simulink model "sliding_car"  (R2017a)
settings: Solver=VariableStepAuto  StartTime=0.0  StopTime=tf  RelTol=1e-3
values from neighbouring files (symbols this model uses):
  a = double(perc*D)    [init_vars.m]
  Cp_1 = 0    [init_vars.m]
  Cp_2 = 0    [init_vars.m]
  Fz_1 = g*(mc/4 + mi)    [init_vars.m]
  Fz_2 = g*(mc/4 + mi)    [init_vars.m]
  mu_1 = 1e-3    (= 0.001)    [init_vars.m]
  mu_2 = 1e-3    (= 0.001)    [init_vars.m]
  x0 = double(subs([qs; ps], [sys.descrip.syms.'; delta_i],                   [sys.descrip.model_params.'; delta_i_num]))    [init_vars.m]    (also in sim_blockdiagram.m)
undefined symbols (not defined in the file or in its folder): g, Ic_33, Ii_11, Ii_21, Ii_22, Ii_31, Ii_32, Ii_33, Il_11, Il_21, Il_22, Il_31, Il_32, Il_33, Io_11, Io_21, Io_22, Io_31, Io_32, Io_33, Ir_11, Ir_21, Ir_22, Ir_31, Ir_32, Ir_33, L, Lc, mc, mi, ml, mo, mr, R, sys, w
(part 1 of 5)
settings Model: SimulationMode=rapid-accelerator  Creator=brunolnetto  LastModifiedBy=brunolnetto

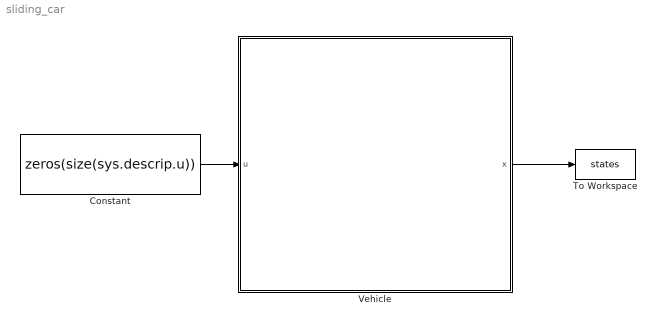
== system sliding_car ==
  Constant : Constant  Value=zeros(size(sys.descrip.u))
  To Workspace : ToWorkspace  VariableName=states  SaveFormat=Structure With Time  SampleTime=-1
  Vehicle : Subsystem
      mask Display: image('/home/brunolnetto/Pictures/auto_model.png');
  wires:
  Constant/1 -> Vehicle/1(u)
  Vehicle/1(x) -> To Workspace/1

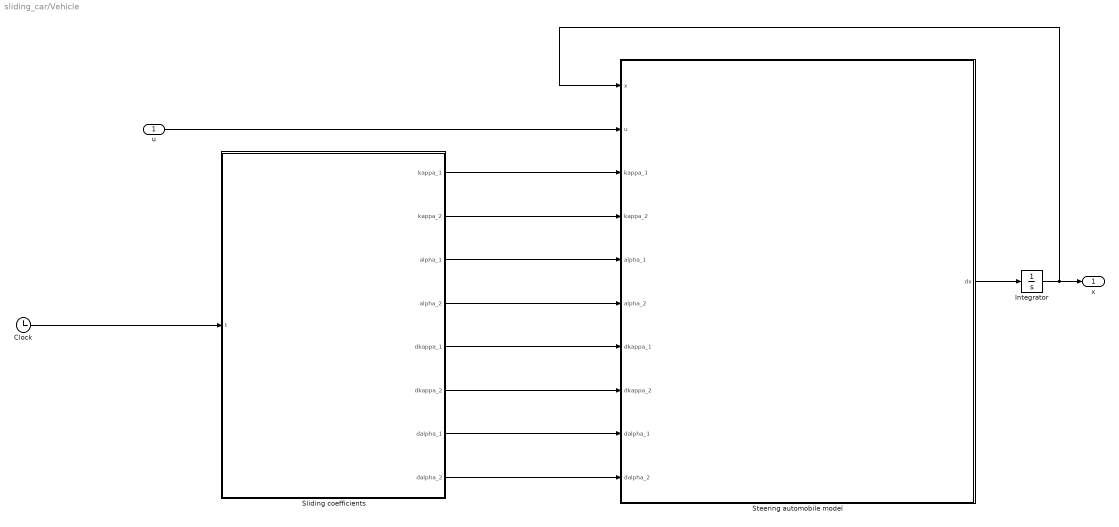
== system sliding_car/Vehicle ==
  u : Inport
  Clock : Clock
  Integrator : Integrator  InitialCondition=x0
  Sliding coefficients : MATLAB Function  TreatAsAtomicUnit=on
  Steering automobile model : Subsystem
      mask Display: image('/home/brunolnetto/Pictures/steer_schema.png');
  x : Outport
  wires:
  Steering automobile model/1(dx) -> Integrator/1
  Sliding coefficients/4(alpha_2) -> Steering automobile model/6(alpha_2)
  Sliding coefficients/3(alpha_1) -> Steering automobile model/5(alpha_1)
  Sliding coefficients/2(kappa_2) -> Steering automobile model/4(kappa_2)
  Sliding coefficients/1(kappa_1) -> Steering automobile model/3(kappa_1)
  u/1 -> Steering automobile model/2(u)
  Clock/1 -> Sliding coefficients/1(t)
  Sliding coefficients/8(dalpha_2) -> Steering automobile model/10(dalpha_2)
  Sliding coefficients/7(dalpha_1) -> Steering automobile model/9(dalpha_1)
  Sliding coefficients/6(dkappa_2) -> Steering automobile model/8(dkappa_2)
  Sliding coefficients/5(dkappa_1) -> Steering automobile model/7(dkappa_1)
  Integrator/1 -> Steering automobile model/1(x), x/1

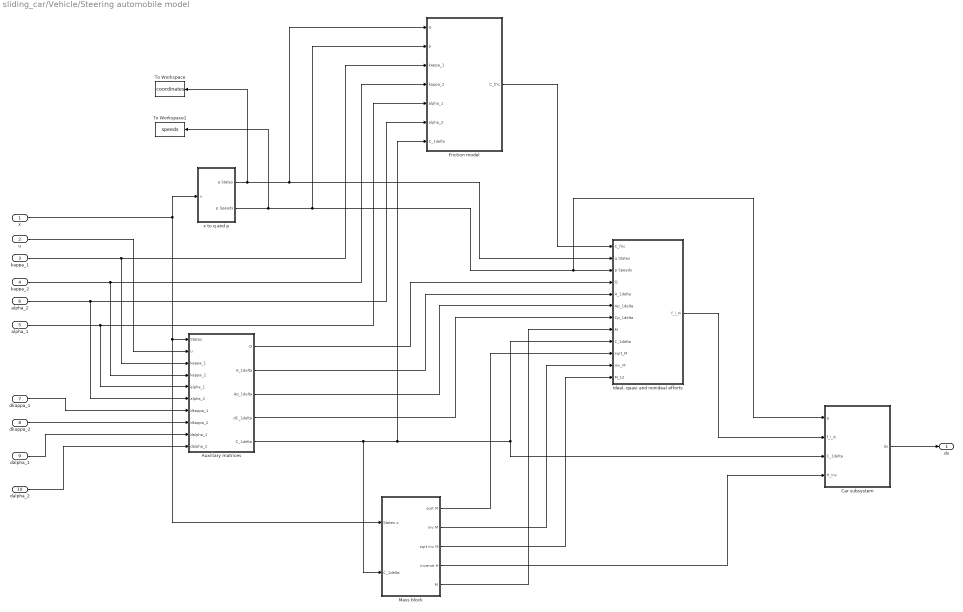
== system sliding_car/Vehicle/Steering automobile model ==
  x : Inport
  u : Inport  Port=2
  kappa_1 : Inport  Port=3
  kappa_2 : Inport  Port=4
  alpha_1 : Inport  Port=5
  alpha_2 : Inport  Port=6
  dkappa_1 : Inport  Port=7
  dkappa_2 : Inport  Port=8
  dalpha_1 : Inport  Port=9
  dalpha_2 : Inport  Port=10
  Auxiliary matrices : Subsystem
  Car subsystem : Subsystem
  Friction model : MATLAB Function  TreatAsAtomicUnit=on
  "Ideal, quasi and nonideal efforts" : Subsystem
  Mass block : Subsystem
  To Workspace : ToWorkspace  VariableName=coordinates  SaveFormat=Structure With Time  SampleTime=-1
  To Workspace1 : ToWorkspace  VariableName=speeds  SaveFormat=Structure With Time  SampleTime=-1
  x to q and p : Subsystem
  dx : Outport
  wires:
  kappa_1/1 -> Auxiliary matrices/3(kappa_1), Friction model/3(kappa_1)
  alpha_2/1 -> Auxiliary matrices/6(alpha_2), Friction model/6(alpha_2)
  alpha_1/1 -> Friction model/5(alpha_1), Auxiliary matrices/5(alpha_1)
  x/1 -> x to q and p/1(x), Mass block/1(States x), Auxiliary matrices/1(States)
  Auxiliary matrices/5("C_1delta ") -> Friction model/7(C_1delta), "Ideal, quasi and nonideal efforts"/9(C_1delta), Car subsystem/3(C_1delta), Mass block/2("C_1delta  ")
  u/1 -> Auxiliary matrices/2(u)
  Auxiliary matrices/1("Q ") -> "Ideal, quasi and nonideal efforts"/4(Q)
  Auxiliary matrices/2("A_1delta ") -> "Ideal, quasi and nonideal efforts"/5(A_1delta)
  Auxiliary matrices/3("Ap_1delta ") -> "Ideal, quasi and nonideal efforts"/6(Ap_1delta)
  Auxiliary matrices/4("dC_1delta ") -> "Ideal, quasi and nonideal efforts"/7(Cp_1delta)
  Mass block/1(sqrt M) -> "Ideal, quasi and nonideal efforts"/10(sqrt_M)
  Mass block/2(inv M) -> "Ideal, quasi and nonideal efforts"/11(inv_M)
  Mass block/3(sqrt inv M) -> "Ideal, quasi and nonideal efforts"/12(M_12)
  dalpha_1/1 -> Auxiliary matrices/9(dalpha_1)
  dkappa_2/1 -> Auxiliary matrices/8(dkappa_2)
  dalpha_2/1 -> Auxiliary matrices/10(dalpha_2)
  dkappa_1/1 -> Auxiliary matrices/7(dkappa_1)
  Mass block/5(M) -> "Ideal, quasi and nonideal efforts"/8(M)
  kappa_2/1 -> Auxiliary matrices/4(kappa_2), Friction model/4(kappa_2)
  Friction model/1(C_fric) -> "Ideal, quasi and nonideal efforts"/1(C_fric)
  Mass block/4(inverse H) -> Car subsystem/4(H_inv)
  Car subsystem/1(dx) -> dx/1
  "Ideal, quasi and nonideal efforts"/1(f_i_ni) -> Car subsystem/2(f_i_ni)
  x to q and p/1(q States) -> Friction model/1(q), "Ideal, quasi and nonideal efforts"/2(q States), To Workspace/1
  x to q and p/2(p Speeds) -> To Workspace1/1, Friction model/2(p), Car subsystem/1(p), "Ideal, quasi and nonideal efforts"/3(p Speeds)

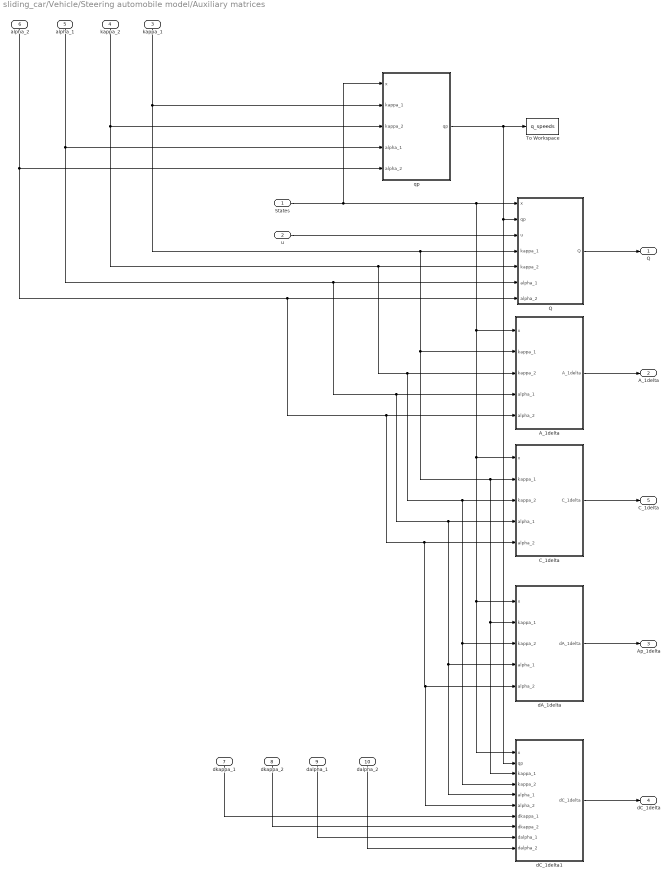
== system sliding_car/Vehicle/Steering automobile model/Auxiliary matrices ==
  States : Inport
  u : Inport  Port=2
  kappa_1 : Inport  Port=3
  kappa_2 : Inport  Port=4
  alpha_1 : Inport  Port=5
  alpha_2 : Inport  Port=6
  dkappa_1 : Inport  Port=7
  dkappa_2 : Inport  Port=8
  dalpha_1 : Inport  Port=9
  dalpha_2 : Inport  Port=10
  A_1delta : MATLAB Function  TreatAsAtomicUnit=on
  C_1delta : MATLAB Function  TreatAsAtomicUnit=on
  Q : MATLAB Function  TreatAsAtomicUnit=on
  To Workspace : ToWorkspace  VariableName=q_speeds  SaveFormat=Structure With Time  SampleTime=-1
  dA_1delta : MATLAB Function  TreatAsAtomicUnit=on
  dC_1delta1 : MATLAB Function  TreatAsAtomicUnit=on
  qp : MATLAB Function  TreatAsAtomicUnit=on
  "Q " : Outport
  "A_1delta " : Outport  Port=2
  "Ap_1delta " : Outport  Port=3
  "dC_1delta " : Outport  Port=4
  "C_1delta " : Outport  Port=5
  wires:
  alpha_2/1 -> Q/7(alpha_2), A_1delta/5(alpha_2), dC_1delta1/6(alpha_2), dA_1delta/5(alpha_2), C_1delta/5(alpha_2), qp/5(alpha_2)
  kappa_2/1 -> Q/5(kappa_2), A_1delta/3(kappa_2), dC_1delta1/4(kappa_2), dA_1delta/3(kappa_2), C_1delta/3(kappa_2), qp/3(kappa_2)
  kappa_1/1 -> A_1delta/2(kappa_1), dC_1delta1/3(kappa_1), dA_1delta/2(kappa_1), C_1delta/2(kappa_1), Q/4(kappa_1), qp/2(kappa_1)
  C_1delta/1(C_1delta) -> "C_1delta "/1
  Q/1(Q) -> "Q "/1
  A_1delta/1(A_1delta) -> "A_1delta "/1
  dC_1delta1/1(dC_1delta) -> "dC_1delta "/1
  dA_1delta/1(dA_1delta) -> "Ap_1delta "/1
  u/1 -> Q/3(u)
  alpha_1/1 -> Q/6(alpha_1), dC_1delta1/5(alpha_1), dA_1delta/4(alpha_1), C_1delta/4(alpha_1), A_1delta/4(alpha_1), qp/4(alpha_1)
  States/1 -> qp/1(x), A_1delta/1(x), dC_1delta1/1(x), dA_1delta/1(x), C_1delta/1(x), Q/1(x)
  qp/1(qp) -> To Workspace/1, dC_1delta1/2(qp), Q/2(qp)
  dalpha_2/1 -> dC_1delta1/10(dalpha_2)
  dalpha_1/1 -> dC_1delta1/9(dalpha_1)
  dkappa_2/1 -> dC_1delta1/8(dkappa_2)
  dkappa_1/1 -> dC_1delta1/7(dkappa_1)

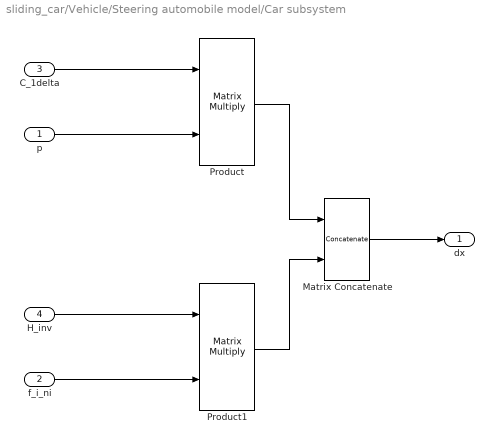
== system sliding_car/Vehicle/Steering automobile model/Car subsystem ==
  p : Inport
  f_i_ni : Inport  Port=2
  C_1delta : Inport  Port=3
  H_inv : Inport  Port=4
  Matrix Concatenate : Concatenate  ConcatenateDimension=2
  Product : Product  Multiplication=Matrix(*)
  Product1 : Product  Multiplication=Matrix(*)
  dx : Outport
  wires:
  Product/1 -> Matrix Concatenate/1
  p/1 -> Product/2
  C_1delta/1 -> Product/1
  Product1/1 -> Matrix Concatenate/2
  H_inv/1 -> Product1/1
  f_i_ni/1 -> Product1/2
  Matrix Concatenate/1 -> dx/1

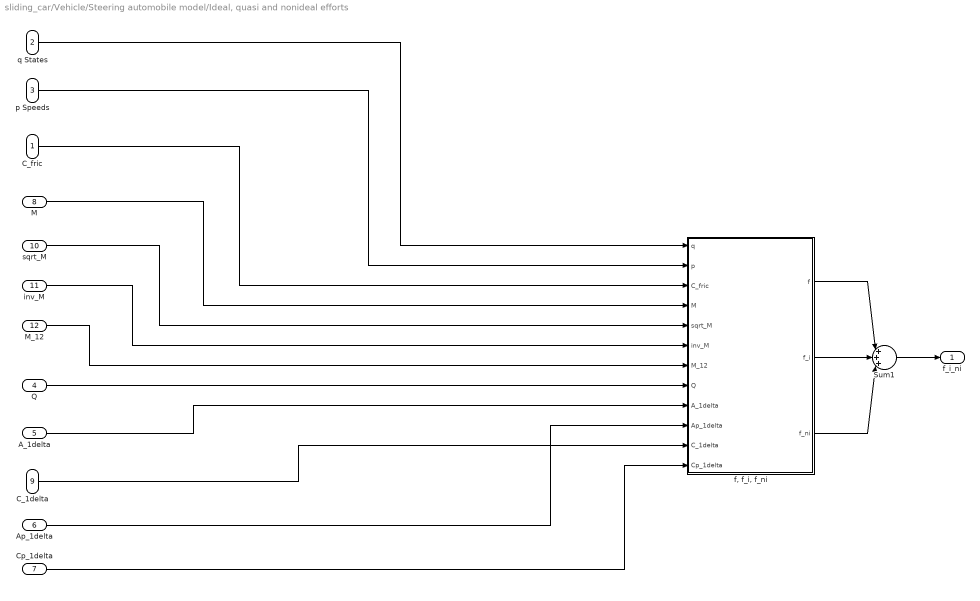
== system sliding_car/Vehicle/Steering automobile model/Ideal, quasi and nonideal efforts ==
  C_fric : Inport
  q States : Inport  Port=2
  p Speeds : Inport  Port=3
  Q : Inport  Port=4
  A_1delta : Inport  Port=5
  Ap_1delta : Inport  Port=6
  Cp_1delta : Inport  Port=7
  M : Inport  Port=8
  C_1delta : Inport  Port=9
  sqrt_M : Inport  Port=10
  inv_M : Inport  Port=11
  M_12 : Inport  Port=12
  Sum1 : Sum  Inputs=|+++|
  "f, f_i, f_ni" : MATLAB Function  TreatAsAtomicUnit=on
  f_i_ni : Outport
  wires:
  inv_M/1 -> "f, f_i, f_ni"/6(inv_M)
  sqrt_M/1 -> "f, f_i, f_ni"/5(sqrt_M)
  M_12/1 -> "f, f_i, f_ni"/7(M_12)
  C_1delta/1 -> "f, f_i, f_ni"/11(C_1delta)
  Q/1 -> "f, f_i, f_ni"/8(Q)
  A_1delta/1 -> "f, f_i, f_ni"/9(A_1delta)
  Cp_1delta/1 -> "f, f_i, f_ni"/12(Cp_1delta)
  Ap_1delta/1 -> "f, f_i, f_ni"/10(Ap_1delta)
  C_fric/1 -> "f, f_i, f_ni"/3(C_fric)
  M/1 -> "f, f_i, f_ni"/4(M)
  q States/1 -> "f, f_i, f_ni"/1(q)
  p Speeds/1 -> "f, f_i, f_ni"/2(p)
  "f, f_i, f_ni"/1(f) -> Sum1/1
  Sum1/1 -> f_i_ni/1
  "f, f_i, f_ni"/2(f_i) -> Sum1/2
  "f, f_i, f_ni"/3(f_ni) -> Sum1/3

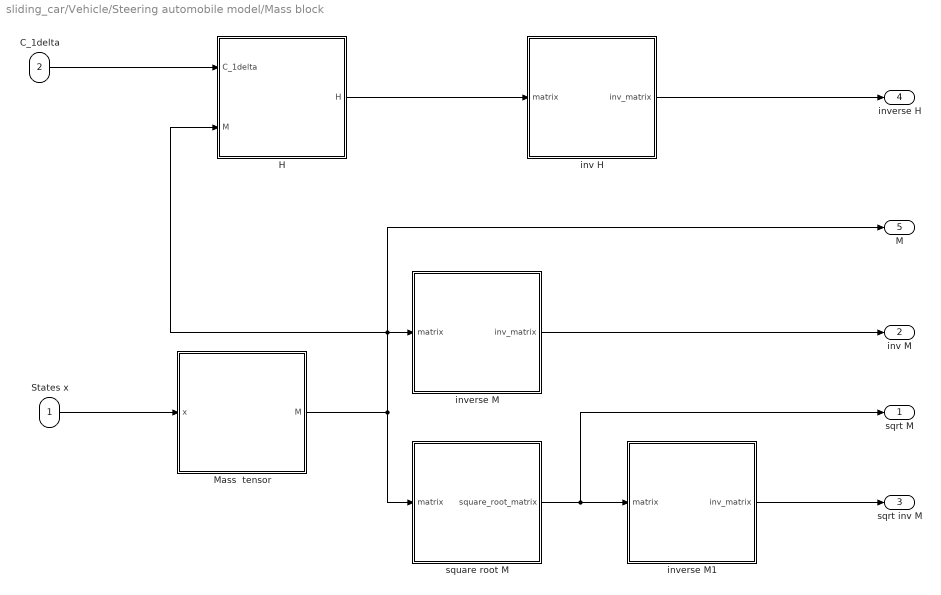
== system sliding_car/Vehicle/Steering automobile model/Mass block ==
  States x : Inport
  "C_1delta  " : Inport  Port=2
  H : MATLAB Function  TreatAsAtomicUnit=on
  Mass  tensor : MATLAB Function  TreatAsAtomicUnit=on
  inv H : MATLAB Function  TreatAsAtomicUnit=on
  inverse M : MATLAB Function  TreatAsAtomicUnit=on
  inverse M1 : MATLAB Function  TreatAsAtomicUnit=on
  square root M : MATLAB Function  TreatAsAtomicUnit=on
  sqrt M : Outport
  inv M : Outport  Port=2
  sqrt inv M : Outport  Port=3
  inverse H : Outport  Port=4
  M : Outport  Port=5
  wires:
  States x/1 -> Mass  tensor/1(x)
  "C_1delta  "/1 -> H/1(C_1delta)
  inverse M/1(inv_matrix) -> inv M/1
  H/1(H) -> inv H/1(matrix)
  inv H/1(inv_matrix) -> inverse H/1
  inverse M1/1(inv_matrix) -> sqrt inv M/1
  Mass  tensor/1(M) -> M/1, H/2(M), inverse M/1(matrix), square root M/1(matrix)
  square root M/1(square_root_matrix) -> sqrt M/1, inverse M1/1(matrix)

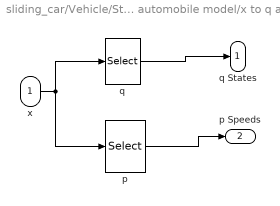
== system sliding_car/Vehicle/Steering automobile model/x to q and p ==
  x : Inport
  p : Selector  InputPortWidth=12  IndexOptions=Index vector (dialog)  Indices=[10 11 12]  OutputSizes=1
  q : Selector  InputPortWidth=12  IndexOptions=Index vector (dialog)  Indices=[1 2 3 4 5 6 7 8 9]  OutputSizes=1
  q States : Outport
  p Speeds : Outport  Port=2
  wires:
  x/1 -> p/1, q/1
  q/1 -> q States/1
  p/1 -> p Speeds/1

== matlab function sliding_car/Vehicle/Steering automobile model/Auxiliary matrices/A_1delta ==
  data: x input; kappa_1 input; kappa_2 input; alpha_1 input; alpha_2 input; w parameter; A_1delta output; L parameter; R parameter
function A_1delta = ConstraintMatrix(x, kappa_1, kappa_2, alpha_1, alpha_2, w, L, R)
%CONSTRAINTMATRIX
%    A_1DELTA = CONSTRAINTMATRIX(L,R,ALPHA_1,ALPHA_2,DELTA_I,DELTA_O,KAPPA_1,KAPPA_2,THETA,W)

%    This function was generated by the Symbolic Math Toolbox version 7.2.
%    16-Oct-2020 13:31:39
    
    x_pos =  x(1);
    y_pos =  x(2);
    theta =  x(3);

    delta_i = x(4);
    delta_o = x(5);

    phi_i = x(6);
    phi_l = x(7);
    phi_o = x(8);
    phi_r = x(9);

    t2 = tan(delta_i);
    t3 = 1.0./L;
    t4 = t2.*w;
    t5 = L+t4;
    t6 = 1.0./t5;
    t7 = t2.*t6;
    t8 = tan(t7);
    t9 = delta_i+theta;
    t10 = cos(t9);
    t11 = sin(t9);
    t12 = tan(alpha_1);
    t13 = cos(delta_i);
    t14 = sin(delta_i);
    t15 = t14.*w.*(1.0./2.0);
    t16 = kappa_1.*t10.*t12;
    t17 = kappa_1.*t11.*t12;
    t18 = kappa_1.*t12.*(t15-L.*t13);
    t19 = L.*t8;
    t20 = atan(t19);
    t21 = t20+theta;
    t22 = delta_o+theta;
    t23 = tan(alpha_2);
    t24 = L.^2;
    t25 = t8.^2;
    t26 = t24.*t25;
    t27 = t26+1.0;
    t28 = 1.0./sqrt(t27);
    t29 = sin(t21);
    t30 = cos(t22);
    t31 = kappa_2.*t23.*t30;
    t32 = cos(t21);
    t33 = sin(t22);
    t34 = kappa_2.*t23.*t33;
    t35 = cos(delta_o);
    t36 = L.*t35;
    t37 = sin(delta_o);
    t38 = t37.*w.*(1.0./2.0);
    t39 = t36+t38;
    A_1delta = reshape([0.0,0.0,t10+t16,-t11+t16,t31+t32,-t29+t31,0.0,0.0, ...
                        t11+t17,t10+t17,t29+t34,t32+t34,0.0,0.0,t15+t18-L.*t13, ...
                        t18+L.*t14+t13.*w.*(1.0./2.0),-L.*t28-kappa_2.*t23.*t39-L.*t8.*t28.*w.*(1.0./2.0), ...
                        t28.*w.*(-1.0./2.0)-kappa_2.*t23.*t39+t8.*t24.*t28,t3.*(t2.^2+1.0).*(L-L.*t8.*w), ...
                        0.0,0.0,0.0,0.0,0.0,-t3.*t5.*t27,0.0,0.0,0.0,0.0,0.0,0.0,0.0,-R,0.0,0.0,0.0, ...
                        0.0,0.0,0.0,0.0,-R,0.0,0.0,-t2.*t3.*w-1.0,0.0,0.0,0.0,0.0,0.0,1.0,0.0,0.0,0.0,0.0],[6,9]);

== matlab function sliding_car/Vehicle/Steering automobile model/Mass block/Mass  tensor ==
  data: x input; M output; Io_32 parameter; Io_33 parameter; Ir_11 parameter; Ir_21 parameter; Ir_22 parameter; Ir_31 parameter; Ir_32 parameter; Ic_33 parameter; Ii_11 parameter; Ii_21 parameter; Ii_22 parameter; Ii_31 parameter; Ii_32 parameter; Ii_33 parameter; Il_11 parameter; Il_21 parameter; Il_22 parameter; Il_31 parameter; Il_32 parameter; Il_33 parameter; Io_11 parameter; Io_21 parameter; Io_22 parameter; Io_31 parameter; Ir_33 parameter; L parameter; Lc parameter; mc parameter; mi parameter; ml parameter; mo parameter; mr parameter; w parameter
function M = MassMatrix(x, ...
                        Io_32, Io_33,...
                        Ir_11, Ir_21, Ir_22, Ir_31, Ir_32, Ic_33, ...
                        Ii_11, Ii_21, Ii_22, Ii_31, Ii_32, Ii_33,...
                        Il_11, Il_21, Il_22, Il_31, Il_32, Il_33,...
                        Io_11, Io_21, Io_22, Io_31, Ir_33,...
                        L, Lc, mc, mi, ml, mo, mr, w)
% MASSMATRIX
%    OUT1 = MASSMATRIX(IC_33,II_11,II_21,II_22,II_31,II_32,II_33,IL_11,IL_21,IL_22,IL_31,IL_32,IL_33,IO_11,IO_21,IO_22,IO_31,IO_32,IO_33,IR_11,IR_21,IR_22,IR_31,IR_32,IR_33,L,LC,DELTA_I,DELTA_O,MC,MI,ML,MO,MR,PHI_I,PHI_L,PHI_O,PHI_R,THETA,W)

%    This function was generated by the Symbolic Math Toolbox version 7.2.
%    16-Oct-2020 11:55:07

x_pos =  x(1);
y_pos =  x(2);
theta =  x(3);

delta_i = x(4);
delta_o = x(5);

phi_i = x(6);
phi_l = x(7);
phi_o = x(8);
phi_r = x(9);

t2 = sin(theta);
t3 = cos(theta);
t4 = mc+mi+ml+mo+mr;
t5 = mo.*t2.*w.*(1.0./2.0);
t6 = mr.*t2.*w.*(1.0./2.0);
t7 = t5+t6-L.*mi.*t3-L.*mo.*t3-Lc.*mc.*t3-mi.*t2.*w.*(1.0./2.0)-ml.*t2.*w.*(1.0./2.0);
t8 = mi.*t3.*w.*(1.0./2.0);
t9 = ml.*t3.*w.*(1.0./2.0);
t10 = t8+t9-L.*mi.*t2-L.*mo.*t2-Lc.*mc.*t2-mo.*t3.*w.*(1.0./2.0)-mr.*t3.*w.*(1.0./2.0);
t11 = cos(phi_i);
t12 = t11.^2;
t13 = cos(phi_l);
t14 = t13.^2;
t15 = cos(phi_o);
t16 = t15.^2;
t17 = cos(phi_r);
t18 = t17.^2;
t19 = sin(phi_l);
t20 = t19.^2;
t21 = t3.^2;
t22 = sin(phi_r);
t23 = t22.^2;
t24 = t2.^2;
t25 = L.^2;
t26 = Lc.^2;
t27 = w.^2;
t28 = t14-1.0;
t29 = t18-1.0;
t30 = cos(delta_i);
t31 = sin(phi_i);
t32 = t31.^2;
t33 = cos(delta_o);
t34 = sin(phi_o);
t35 = t34.^2;
t36 = t30.^2;
t37 = sin(delta_i);
t38 = t33.^2;
t39 = sin(delta_o);
t40 = t37.^2;
t41 = t32.^2;
t42 = t39.^2;
t43 = t35.^2;
t44 = phi_i.*4.0;
t45 = cos(t44);
t46 = t45-1.0;
t47 = t12.^2;
t48 = Ii_33.*t47;
t49 = Ii_33.*t21.*t36.*t41;
t50 = Ii_22.*t24.*t32.*t36;
t51 = Ii_22.*t21.*t32.*t40;
t52 = Ii_33.*t24.*t40.*t41;
t53 = Ii_31.*t11.*t21.*t31.*t32.*t36.*2.0;
t54 = Ii_31.*t11.*t24.*t31.*t32.*t40.*2.0;
t55 = Ii_31.*t3.*t11.*t30.*t31.*t32.*2.0;
t56 = Ii_32.*t2.*t12.*t30.*t31.*2.0;
t57 = Ii_32.*t3.*t12.*t31.*t37.*2.0;
t58 = Ii_11.*t12.*t21.*t32.*t36;
t59 = Ii_31.*t2.*t11.*t12.*t31.*t37.*2.0;
t60 = Ii_11.*t12.*t24.*t32.*t40;
t61 = Ii_11.*t3.*t12.*t30.*t32.*2.0;
t62 = Ii_32.*t24.*t30.*t31.*t32.*t37.*2.0;
t63 = Ii_33.*t2.*t12.*t32.*t37.*2.0;
t64 = Ii_32.*t2.*t3.*t31.*t32.*t40.*2.0;
t65 = Ii_22.*t2.*t3.*t30.*t32.*t37.*2.0;
t66 = Ii_21.*t11.*t24.*t30.*t32.*t37.*2.0;
t67 = Ii_21.*t2.*t3.*t11.*t32.*t40.*2.0;
t68 = phi_o.*4.0;
t69 = cos(t68);
t70 = t69-1.0;
t71 = t16.^2;
t72 = Io_33.*t71;
t73 = Io_33.*t21.*t38.*t43;
t74 = Io_22.*t24.*t35.*t38;
t75 = Io_22.*t21.*t35.*t42;
t76 = Io_33.*t24.*t42.*t43;
t77 = Io_31.*t15.*t21.*t34.*t35.*t38.*2.0;
t78 = Io_31.*t15.*t24.*t34.*t35.*t42.*2.0;
t79 = Io_31.*t3.*t15.*t33.*t34.*t35.*2.0;
t80 = Io_32.*t2.*t16.*t33.*t34.*2.0;
t81 = Io_32.*t3.*t16.*t34.*t39.*2.0;
t82 = Io_11.*t16.*t21.*t35.*t38;
t83 = Io_31.*t2.*t15.*t16.*t34.*t39.*2.0;
t84 = Io_11.*t16.*t24.*t35.*t42;
t85 = Io_11.*t3.*t16.*t33.*t35.*2.0;
t86 = Io_32.*t24.*t33.*t34.*t35.*t39.*2.0;
t87 = Io_33.*t2.*t16.*t35.*t39.*2.0;
t88 = Io_32.*t2.*t3.*t34.*t35.*t42.*2.0;
t89 = Io_22.*t2.*t3.*t33.*t35.*t39.*2.0;
t90 = Io_21.*t15.*t24.*t33.*t35.*t39.*2.0;
t91 = Io_21.*t2.*t3.*t15.*t35.*t42.*2.0;
t92 = delta_i.*2.0;
t93 = theta.*2.0;
t94 = cos(t92);
t95 = cos(t93);
t96 = phi_i.*2.0;
t97 = sin(t93);
t98 = phi_i.*3.0;
t99 = cos(t98);
t100 = sin(t92);
t101 = sin(t98);
t102 = cos(t96);
t103 = sin(t96);
t104 = delta_o.*2.0;
t105 = cos(t104);
t106 = phi_o.*2.0;
t107 = phi_o.*3.0;
t108 = cos(t107);
t109 = sin(t104);
t110 = sin(t107);
t111 = cos(t106);
t112 = sin(t106);
t114 = Ii_11.*t46.*(1.0./8.0);
t115 = Ii_31.*t11.*t12.*t31.*2.0;
t116 = Ii_31.*t3.*t11.*t12.*t30.*t31.*2.0;
t117 = Ii_21.*t2.*t11.*t30.*t32.*2.0;
t118 = Ii_21.*t3.*t11.*t32.*t37.*2.0;
t119 = Ii_31.*t2.*t11.*t31.*t32.*t37.*2.0;
t120 = Ii_33.*t3.*t12.*t30.*t32.*2.0;
t121 = Ii_32.*t21.*t30.*t31.*t32.*t37.*2.0;
t122 = Ii_32.*t2.*t3.*t31.*t32.*t36.*2.0;
t123 = Ii_11.*t2.*t12.*t32.*t37.*2.0;
t124 = Ii_33.*t2.*t3.*t30.*t37.*t41.*2.0;
t125 = Ii_21.*t11.*t21.*t30.*t32.*t37.*2.0;
t126 = Ii_21.*t2.*t3.*t11.*t32.*t36.*2.0;
t127 = Ii_31.*t2.*t3.*t11.*t30.*t31.*t32.*t37.*4.0;
t128 = Ii_11.*t2.*t3.*t12.*t30.*t32.*t37.*2.0;
t113 = t48+t49+t50+t51+t52+t53+t54+t55+t56+t57+t58+t59+t60+t61+t62+t63+t64+t65+t66+t67-t114-t115-t116-t117-t118-t119-t120-t121-t122-t123-t124-t125-t126-t127-t128;
t129 = Ii_32.*t97.*t100.*(1.0./2.0);
t130 = Ii_32.*t3.*t30.*(1.0./2.0);
t131 = Ii_31.*t2.*t11.*t30.*(1.0./2.0);
t132 = Ii_31.*t3.*t11.*t37.*(1.0./2.0);
t133 = Ii_32.*t94.*t95.*t102.*(1.0./2.0);
t134 = Ii_33.*t2.*t30.*t31.*(1.0./4.0);
t135 = Ii_33.*t3.*t31.*t37.*(1.0./4.0);
t136 = Ii_31.*t94.*t97.*t99.*(1.0./4.0);
t137 = Ii_31.*t95.*t99.*t100.*(1.0./4.0);
t138 = Ii_33.*t94.*t97.*t101.*(1.0./8.0);
t139 = Ii_33.*t95.*t100.*t101.*(1.0./8.0);
t140 = Ii_21.*t97.*t100.*t103.*(1.0./2.0);
t141 = Ii_32.*t3.*t30.*t102.*(1.0./2.0);
t142 = Ii_31.*t2.*t30.*t99.*(1.0./2.0);
t143 = Ii_31.*t3.*t37.*t99.*(1.0./2.0);
t144 = Ii_33.*t2.*t30.*t101.*(1.0./4.0);
t145 = Ii_33.*t3.*t37.*t101.*(1.0./4.0);
t146 = Ii_21.*t2.*t37.*t103.*(1.0./2.0);
t147 = Ii_22.*t31.*t94.*t97.*(1.0./2.0);
t148 = Ii_22.*t31.*t95.*t100.*(1.0./2.0);
t187 = Ii_32.*t94.*t95.*(1.0./2.0);
t188 = Ii_32.*t2.*t37.*(1.0./2.0);
t189 = Ii_11.*t2.*t30.*t31.*(1.0./4.0);
t190 = Ii_11.*t3.*t31.*t37.*(1.0./4.0);
t191 = Ii_21.*t94.*t95.*t103.*(1.0./2.0);
t192 = Ii_11.*t94.*t97.*t101.*(1.0./8.0);
t193 = Ii_11.*t95.*t100.*t101.*(1.0./8.0);
t194 = Ii_32.*t97.*t100.*t102.*(1.0./2.0);
t195 = Ii_21.*t3.*t30.*t103.*(1.0./2.0);
t196 = Ii_11.*t2.*t30.*t101.*(1.0./4.0);
t197 = Ii_11.*t3.*t37.*t101.*(1.0./4.0);
t198 = Ii_32.*t2.*t37.*t102.*(1.0./2.0);
t199 = Ii_31.*t11.*t94.*t97.*(1.0./4.0);
t200 = Ii_31.*t11.*t95.*t100.*(1.0./4.0);
t201 = Ii_11.*t31.*t94.*t97.*(1.0./8.0);
t202 = Ii_11.*t31.*t95.*t100.*(1.0./8.0);
t203 = Ii_33.*t31.*t94.*t97.*(3.0./8.0);
t204 = Ii_33.*t31.*t95.*t100.*(3.0./8.0);
t149 = t129+t130+t131+t132+t133+t134+t135+t136+t137+t138+t139+t140+t141+t142+t143+t144+t145+t146+t147+t148-t187-t188-t189-t190-t191-t192-t193-t194-t195-t196-t197-t198-t199-t200-t201-t202-t203-t204;
t151 = Io_11.*t70.*(1.0./8.0);
t152 = Io_31.*t15.*t16.*t34.*2.0;
t153 = Io_31.*t3.*t15.*t16.*t33.*t34.*2.0;
t154 = Io_21.*t2.*t15.*t33.*t35.*2.0;
t155 = Io_21.*t3.*t15.*t35.*t39.*2.0;
t156 = Io_31.*t2.*t15.*t34.*t35.*t39.*2.0;
t157 = Io_33.*t3.*t16.*t33.*t35.*2.0;
t158 = Io_32.*t21.*t33.*t34.*t35.*t39.*2.0;
t159 = Io_32.*t2.*t3.*t34.*t35.*t38.*2.0;
t160 = Io_11.*t2.*t16.*t35.*t39.*2.0;
t161 = Io_33.*t2.*t3.*t33.*t39.*t43.*2.0;
t162 = Io_21.*t15.*t21.*t33.*t35.*t39.*2.0;
t163 = Io_21.*t2.*t3.*t15.*t35.*t38.*2.0;
t164 = Io_31.*t2.*t3.*t15.*t33.*t34.*t35.*t39.*4.0;
t165 = Io_11.*t2.*t3.*t16.*t33.*t35.*t39.*2.0;
t150 = t72+t73+t74+t75+t76+t77+t78+t79+t80+t81+t82+t83+t84+t85+t86+t87+t88+t89+t90+t91-t151-t152-t153-t154-t155-t156-t157-t158-t159-t160-t161-t162-t163-t164-t165;
t166 = Io_32.*t97.*t109.*(1.0./2.0);
t167 = Io_32.*t3.*t33.*(1.0./2.0);
t168 = Io_31.*t2.*t15.*t33.*(1.0./2.0);
t169 = Io_31.*t3.*t15.*t39.*(1.0./2.0);
t170 = Io_32.*t95.*t105.*t111.*(1.0./2.0);
t171 = Io_33.*t2.*t33.*t34.*(1.0./4.0);
t172 = Io_33.*t3.*t34.*t39.*(1.0./4.0);
t173 = Io_31.*t97.*t105.*t108.*(1.0./4.0);
t174 = Io_31.*t95.*t108.*t109.*(1.0./4.0);
t175 = Io_33.*t97.*t105.*t110.*(1.0./8.0);
t176 = Io_33.*t95.*t109.*t110.*(1.0./8.0);
t177 = Io_21.*t97.*t109.*t112.*(1.0./2.0);
t178 = Io_32.*t3.*t33.*t111.*(1.0./2.0);
t179 = Io_31.*t2.*t33.*t108.*(1.0./2.0);
t180 = Io_31.*t3.*t39.*t108.*(1.0./2.0);
t181 = Io_33.*t2.*t33.*t110.*(1.0./4.0);
t182 = Io_33.*t3.*t39.*t110.*(1.0./4.0);
t183 = Io_21.*t2.*t39.*t112.*(1.0./2.0);
t184 = Io_22.*t34.*t97.*t105.*(1.0./2.0);
t185 = Io_22.*t34.*t95.*t109.*(1.0./2.0);
t205 = Io_32.*t95.*t105.*(1.0./2.0);
t206 = Io_32.*t2.*t39.*(1.0./2.0);
t207 = Io_11.*t2.*t33.*t34.*(1.0./4.0);
t208 = Io_11.*t3.*t34.*t39.*(1.0./4.0);
t209 = Io_21.*t95.*t105.*t112.*(1.0./2.0);
t210 = Io_11.*t97.*t105.*t110.*(1.0./8.0);
t211 = Io_11.*t95.*t109.*t110.*(1.0./8.0);
t212 = Io_32.*t97.*t109.*t111.*(1.0./2.0);
t213 = Io_21.*t3.*t33.*t112.*(1.0./2.0);
t214 = Io_11.*t2.*t33.*t110.*(1.0./4.0);
t215 = Io_11.*t3.*t39.*t110.*(1.0./4.0);
t216 = Io_32.*t2.*t39.*t111.*(1.0./2.0);
t217 = Io_31.*t15.*t97.*t105.*(1.0./4.0);
t218 = Io_31.*t15.*t95.*t109.*(1.0./4.0);
t219 = Io_11.*t34.*t97.*t105.*(1.0./8.0);
t220 = Io_11.*t34.*t95.*t109.*(1.0./8.0);
t221 = Io_33.*t34.*t97.*t105.*(3.0./8.0);
t222 = Io_33.*t34.*t95.*t109.*(3.0./8.0);
t186 = t166+t167+t168+t169+t170+t171+t172+t173+t174+t175+t176+t177+t178+t179+t180+t181+t182+t183+t184+t185-t205-t206-t207-t208-t209-t210-t211-t212-t213-t214-t215-t216-t217-t218-t219-t220-t221-t222;
t223 = Ir_32.*t23.*t24;
t224 = Ir_32.*t3.*t18;
t225 = Ir_31.*t2.*t17.*t18;
t226 = Ir_22.*t2.*t3.*t22;
t227 = Ir_21.*t17.*t22.*t24;
t228 = Ir_33.*t2.*t18.*t22;
t229 = t223+t224+t225+t226+t227+t228-Ir_32.*t21.*t23-Ir_11.*t2.*t18.*t22-Ir_21.*t3.*t17.*t22-Ir_31.*t2.*t17.*t23-Ir_21.*t17.*t21.*t22-Ir_11.*t2.*t3.*t18.*t22-Ir_31.*t2.*t3.*t17.*t23.*2.0-Ir_33.*t2.*t3.*t22.*t23;
t230 = Il_32.*t20.*t24;
t231 = Il_32.*t3.*t14;
t232 = Il_31.*t2.*t13.*t14;
t233 = Il_22.*t2.*t3.*t19;
t234 = Il_21.*t13.*t19.*t24;
t235 = Il_33.*t2.*t14.*t19;
t236 = t230+t231+t232+t233+t234+t235-Il_32.*t20.*t21-Il_11.*t2.*t14.*t19-Il_21.*t3.*t13.*t19-Il_31.*t2.*t13.*t20-Il_21.*t13.*t19.*t21-Il_11.*t2.*t3.*t14.*t19-Il_31.*t2.*t3.*t13.*t20.*2.0-Il_33.*t2.*t3.*t19.*t20;
M = reshape([t4,0.0,t7,0.0,0.0,0.0,0.0,0.0,0.0,0.0,t4,t10,0.0,0.0,0.0,0.0,0.0,0.0,t7,t10,Ic_33+t48+t49+t50+t51+t52+t53+t54+t55+t56+t57+t58+t59+t60+t61+t62+t63+t64+t65+t66+t67+t72+t73+t74+t75+t76+t77+t78+t79+t80+t81+t82+t83+t84+t85+t86+t87+t88+t89+t90+t91-Ii_11.*t46.*(1.0./8.0)-Io_11.*t70.*(1.0./8.0)-Il_11.*(cos(phi_l.*4.0)-1.0).*(1.0./8.0)-Ir_11.*(cos(phi_r.*4.0)-1.0).*(1.0./8.0)+Il_33.*t14.^2+Ir_33.*t18.^2+Il_22.*t20.*t24+Ir_22.*t23.*t24+mc.*t21.*t26+mc.*t24.*t26+mi.*t21.*t25+mi.*t21.*t27.*(1.0./4.0)+mi.*t24.*t25+mi.*t24.*t27.*(1.0./4.0)+ml.*t21.*t27.*(1.0./4.0)+ml.*t24.*t27.*(1.0./4.0)+mo.*t21.*t25+mo.*t21.*t27.*(1.0./4.0)+mo.*t24.*t25+mo.*t24.*t27.*(1.0./4.0)+mr.*t21.*t27.*(1.0./4.0)+mr.*t24.*t27.*(1.0./4.0)+Il_33.*t20.^2.*t21+Ir_33.*t21.*t23.^2-Ii_31.*t11.*t12.*t31.*2.0-Il_11.*t3.*t14.*t28.*2.0+Il_21.*t2.*t13.*t28.*2.0+Il_11.*t14.*t20.*t21-Il_31.*t13.*t14.*t19.*2.0+Il_33.*t3.*t14.*t28.*2.0-Io_31.*t15.*t16.*t34.*2.0-Ir_11.*t3.*t18.*t29.*2.0+Ir_21.*t2.*t17.*t29.*2.0+Ir_11.*t18.*t21.*t23+Ir_33.*t3.*t18.*t29.*2.0-Ir_31.*t17.*t18.*t22.*2.0-Il_32.*t2.*t19.*(t20-1.0).*2.0-Ir_32.*t2.*t22.*(t23-1.0).*2.0-Ii_11.*t2.*t12.*t32.*t37.*2.0-Ii_21.*t2.*t11.*t30.*t32.*2.0-Ii_21.*t3.*t11.*t32.*t37.*2.0-Ii_33.*t3.*t12.*t30.*t32.*2.0-Il_21.*t2.*t3.*t13.*t20.*2.0-Il_32.*t2.*t3.*t19.*t20.*2.0-Il_31.*t3.*t13.*t14.*t19.*2.0+Il_31.*t3.*t13.*t19.*t20.*2.0+Il_31.*t13.*t19.*t20.*t21.*2.0-Io_11.*t2.*t16.*t35.*t39.*2.0-Io_21.*t2.*t15.*t33.*t35.*2.0-Io_21.*t3.*t15.*t35.*t39.*2.0-Io_33.*t3.*t16.*t33.*t35.*2.0-Ir_21.*t2.*t3.*t17.*t23.*2.0-Ir_32.*t2.*t3.*t22.*t23.*2.0-Ir_31.*t3.*t17.*t18.*t22.*2.0+Ir_31.*t3.*t17.*t22.*t23.*2.0+Ir_31.*t17.*t21.*t22.*t23.*2.0-Ii_21.*t2.*t3.*t11.*t32.*t36.*2.0-Ii_31.*t3.*t11.*t12.*t30.*t31.*2.0-Ii_32.*t2.*t3.*t31.*t32.*t36.*2.0-Ii_31.*t2.*t11.*t31.*t32.*t37.*2.0-Ii_33.*t2.*t3.*t30.*t37.*t41.*2.0-Ii_21.*t11.*t21.*t30.*t32.*t37.*2.0-Ii_32.*t21.*t30.*t31.*t32.*t37.*2.0-Io_21.*t2.*t3.*t15.*t35.*t38.*2.0-Io_31.*t3.*t15.*t16.*t33.*t34.*2.0-Io_32.*t2.*t3.*t34.*t35.*t38.*2.0-Io_33.*t2.*t3.*t33.*t39.*t43.*2.0-Io_31.*t2.*t15.*t34.*t35.*t39.*2.0-Io_21.*t15.*t21.*t33.*t35.*t39.*2.0-Io_32.*t21.*t33.*t34.*t35.*t39.*2.0-Ii_11.*t2.*t3.*t12.*t30.*t32.*t37.*2.0-Io_11.*t2.*t3.*t16.*t33.*t35.*t39.*2.0-Ii_31.*t2.*t3.*t11.*t30.*t31.*t32.*t37.*4.0-Io_31.*t2.*t3.*t15.*t33.*t34.*t35.*t39.*4.0,t113,t150,t149,t186,t229,t236,0.0,0.0,t113,t113,0.0,t149,0.0,0.0,0.0,0.0,0.0,t150,0.0,t150,0.0,t186,0.0,0.0,0.0,0.0,t149,t149,0.0,Ii_22.*(1.0./2.0)+Ii_33.*(1.0./2.0)+Ii_11.*t12.*(1.0./2.0)-Ii_33.*t12.*(1.0./2.0)+Ii_31.*t103.*(1.0./2.0)+Ii_22.*t94.*t95.*(1.0./2.0)-Ii_22.*t97.*t100.*(1.0./2.0)-Ii_33.*t94.*t95.*(1.0./2.0)+Ii_33.*t97.*t100.*(1.0./2.0)-Ii_11.*t12.*t94.*t95.*(1.0./2.0)+Ii_11.*t12.*t97.*t100.*(1.0./2.0)+Ii_21.*t11.*t94.*t97+Ii_21.*t11.*t95.*t100+Ii_33.*t12.*t94.*t95.*(1.0./2.0)-Ii_33.*t12.*t97.*t100.*(1.0./2.0)+Ii_32.*t31.*t94.*t97+Ii_32.*t31.*t95.*t100-Ii_31.*t11.*t31.*t94.*t95+Ii_31.*t11.*t31.*t97.*t100,0.0,0.0,0.0,0.0,0.0,t186,0.0,t186,0.0,Io_22.*(1.0./2.0)+Io_33.*(1.0./2.0)+Io_11.*t16.*(1.0./2.0)-Io_33.*t16.*(1.0./2.0)+Io_31.*t112.*(1.0./2.0)+Io_22.*t95.*t105.*(1.0./2.0)-Io_22.*t97.*t109.*(1.0./2.0)-Io_33.*t95.*t105.*(1.0./2.0)+Io_33.*t97.*t109.*(1.0./2.0)-Io_11.*t16.*t95.*t105.*(1.0./2.0)+Io_11.*t16.*t97.*t109.*(1.0./2.0)+Io_21.*t15.*t97.*t105+Io_21.*t15.*t95.*t109+Io_33.*t16.*t95.*t105.*(1.0./2.0)-Io_33.*t16.*t97.*t109.*(1.0./2.0)+Io_32.*t34.*t97.*t105+Io_32.*t34.*t95.*t109-Io_31.*t15.*t34.*t95.*t105+Io_31.*t15.*t34.*t97.*t109,0.0,0.0,0.0,0.0,t229,0.0,0.0,0.0,0.0,Ir_22.*t21+Ir_11.*t18.*t24+Ir_33.*t23.*t24+Ir_21.*t2.*t3.*t17.*2.0+Ir_32.*t2.*t3.*t22.*2.0+Ir_31.*t17.*t22.*t24.*2.0,0.0,0.0,0.0,t236,0.0,0.0,0.0,0.0,0.0,Il_22.*t21+Il_11.*t14.*t24+Il_33.*t20.*t24+Il_21.*t2.*t3.*t13.*2.0+Il_32.*t2.*t3.*t19.*2.0+Il_31.*t13.*t19.*t24.*2.0],[9,9]);

== matlab function sliding_car/Vehicle/Steering automobile model/Auxiliary matrices/C_1delta ==
  data: x input; kappa_1 input; kappa_2 input; alpha_1 input; alpha_2 input; L parameter; R parameter; w parameter; C_1delta output
function C_1delta = KinematicMatrix(x, kappa_1, kappa_2, alpha_1, alpha_2, L, R, w)
%KINEMATICMATRIX
%    C_1DELTA = KINEMATICMATRIX(L,R,ALPHA_1,ALPHA_2,DELTA_I,DELTA_O,KAPPA_1,KAPPA_2,THETA,W)

%    This function was generated by the Symbolic Math Toolbox version 7.2.
%    16-Oct-2020 13:31:27

    x_pos =  x(1);
    y_pos =  x(2);
    theta =  x(3);

    delta_i = x(4);
    delta_o = x(5);

    phi_i = x(6);
    phi_l = x(7);
    phi_o = x(8);
    phi_r = x(9);

    t2 = tan(delta_i);
    t3 = delta_i+theta;
    t4 = cos(t3);
    t5 = t2.*w;
    t6 = L+t5;
    t7 = 1.0./t6;
    t8 = t2.*t7;
    t9 = tan(t8);
    t10 = L.^2;
    t11 = L.*t9;
    t12 = atan(t11);
    t13 = t12+theta;
    t14 = cos(t13);
    t15 = t9.^2;
    t16 = t10.*t15;
    t17 = t16+1.0;
    t18 = sqrt(t17);
    t19 = sin(t3);
    t20 = tan(alpha_1);
    t21 = cos(delta_i);
    t22 = tan(alpha_2);
    t23 = sin(delta_i);
    t24 = delta_o+theta;
    t25 = sin(t24);
    t26 = cos(delta_o);
    t27 = sin(delta_o);
    t28 = sin(t13);
    t29 = t14.^2;
    t30 = t28.^2;
    t31 = cos(t24);
    t32 = L.*t4.*t28.*2.0;
    t33 = t4.*t14.*w;
    t34 = t19.*t28.*w;
    t35 = L.*t18.*t23.*t29.*2.0;
    t36 = L.*t18.*t23.*t30.*2.0;
    t37 = t18.*t21.*t29.*w;
    t38 = t18.*t21.*t30.*w;
    t39 = L.*kappa_1.*t4.*t14.*t20.*2.0;
    t40 = kappa_2.*t4.*t22.*t31.*w;
    t41 = L.*kappa_1.*t19.*t20.*t28.*2.0;
    t42 = kappa_1.*t14.*t19.*t20.*w;
    t43 = kappa_2.*t19.*t22.*t25.*w;
    t44 = L.*t4.*t9.*t28.*w;
    t45 = kappa_1.*t4.*t9.*t10.*t20.*t28.*2.0;
    t46 = kappa_1.*t18.*t20.*t23.*t29.*w;
    t47 = kappa_1.*t18.*t20.*t23.*t30.*w;
    t48 = L.*kappa_1.*t4.*t9.*t14.*t20.*w;
    t49 = L.*kappa_1.*t9.*t19.*t20.*t28.*w;
    t50 = L.*kappa_1.*kappa_2.*t4.*t20.*t22.*t25.*2.0;
    t51 = L.*kappa_2.*t4.*t14.*t18.*t22.*t26.*2.0;
    t52 = L.*kappa_2.*t4.*t18.*t22.*t26.*t28.*2.0;
    t53 = L.*kappa_2.*t14.*t18.*t22.*t23.*t31.*2.0;
    t54 = kappa_1.*kappa_2.*t19.*t20.*t22.*t31.*w;
    t55 = L.*kappa_2.*t14.*t18.*t22.*t23.*t25.*2.0;
    t56 = L.*kappa_2.*t18.*t19.*t22.*t26.*t28.*2.0;
    t57 = kappa_2.*t14.*t18.*t21.*t22.*t31.*w;
    t58 = L.*kappa_2.*t18.*t22.*t23.*t25.*t28.*2.0;
    t59 = kappa_2.*t4.*t14.*t18.*t22.*t27.*w;
    t60 = kappa_2.*t14.*t18.*t21.*t22.*t25.*w;
    t61 = kappa_2.*t4.*t18.*t22.*t27.*t28.*w;
    t62 = kappa_2.*t18.*t21.*t22.*t25.*t28.*w;
    t63 = kappa_2.*t18.*t19.*t22.*t27.*t28.*w;
    t64 = kappa_1.*kappa_2.*t4.*t9.*t10.*t20.*t22.*t25.*2.0;
    t65 = kappa_1.*kappa_2.*t4.*t14.*t18.*t20.*t22.*t27.*w;
    t66 = kappa_1.*kappa_2.*t14.*t18.*t20.*t22.*t23.*t31.*w;
    t67 = kappa_1.*kappa_2.*t14.*t18.*t19.*t20.*t22.*t27.*w;
    t68 = kappa_1.*kappa_2.*t14.*t18.*t20.*t22.*t23.*t25.*w;
    t69 = kappa_1.*kappa_2.*t18.*t19.*t20.*t22.*t27.*t28.*w;
    t70 = kappa_1.*kappa_2.*t18.*t20.*t22.*t23.*t25.*t28.*w;
    t71 = L.*kappa_1.*kappa_2.*t4.*t9.*t20.*t22.*t25.*w;
    t72 = L.*kappa_1.*kappa_2.*t4.*t14.*t18.*t20.*t22.*t26.*2.0;
    t73 = L.*kappa_1.*kappa_2.*t18.*t20.*t21.*t22.*t28.*t31.*2.0;
    t74 = L.*kappa_1.*kappa_2.*t14.*t18.*t19.*t20.*t22.*t26.*2.0;
    t75 = L.*kappa_1.*kappa_2.*t18.*t19.*t20.*t22.*t26.*t28.*2.0;
    t78 = L.*t14.*t19.*2.0;
    t79 = t4.*t9.*t10.*t14.*2.0;
    t80 = t9.*t10.*t19.*t28.*2.0;
    t81 = L.*kappa_2.*t4.*t22.*t31.*2.0;
    t82 = L.*kappa_2.*t19.*t22.*t25.*2.0;
    t83 = kappa_1.*t4.*t20.*t28.*w;
    t84 = L.*t9.*t14.*t19.*w;
    t85 = kappa_1.*t9.*t10.*t14.*t19.*t20.*2.0;
    t86 = kappa_2.*t9.*t10.*t19.*t22.*t25.*2.0;
    t87 = L.*kappa_1.*t18.*t20.*t21.*t29.*2.0;
    t88 = L.*kappa_1.*t18.*t20.*t21.*t30.*2.0;
    t89 = kappa_2.*t4.*t9.*t10.*t22.*t31.*2.0;
    t90 = L.*kappa_2.*t4.*t9.*t22.*t31.*w;
    t91 = L.*kappa_2.*t9.*t19.*t22.*t25.*w;
    t92 = L.*kappa_1.*kappa_2.*t19.*t20.*t22.*t31.*2.0;
    t93 = L.*kappa_2.*t14.*t18.*t19.*t22.*t26.*2.0;
    t94 = kappa_1.*kappa_2.*t4.*t20.*t22.*t25.*w;
    t95 = L.*kappa_2.*t18.*t22.*t23.*t28.*t31.*2.0;
    t96 = kappa_2.*t18.*t21.*t22.*t28.*t31.*w;
    t97 = kappa_2.*t14.*t18.*t19.*t22.*t27.*w;
    t98 = kappa_1.*kappa_2.*t9.*t10.*t19.*t20.*t22.*t31.*2.0;
    t99 = kappa_1.*kappa_2.*t4.*t18.*t20.*t22.*t27.*t28.*w;
    t100 = kappa_1.*kappa_2.*t18.*t20.*t22.*t23.*t28.*t31.*w;
    t101 = L.*kappa_1.*kappa_2.*t9.*t19.*t20.*t22.*t31.*w;
    t102 = L.*kappa_1.*kappa_2.*t14.*t18.*t20.*t21.*t22.*t31.*2.0;
    t103 = L.*kappa_1.*kappa_2.*t4.*t18.*t20.*t22.*t26.*t28.*2.0;
    t104 = L.*kappa_1.*kappa_2.*t14.*t18.*t20.*t21.*t22.*t25.*2.0;
    t105 = L.*kappa_1.*kappa_2.*t18.*t20.*t21.*t22.*t25.*t28.*2.0;
    t76 = t32+t33+t34+t35+t36+t37+t38+t39+t40+t41+t42+t43+t44+t45+t46+t47+t48+t49+t50+...
          t51+t52+t53+t54+t55+t56+t57+t58+t59+t60+t61+t62+t63+t64+t65+t66+t67+t68+t69+...
          t70+t71+t72+t73+t74+t75-t78-t79-t80-t81-t82-t83-t84-t85-t86-t87-t88-t89-t90-...
          t91-t92-t93-t94-t95-t96-t97-t98-t99-t100-t101-t102-t103-t104-t105;
    t77 = 1.0./t76;
    t106 = t4.^2;
    t107 = t19.^2;
    C_1delta = reshape([0.0,0.0,0.0,-(t6.*t17)./(L.*(t2.^2+1.0).*(t9.*w-1.0)),...
                        1.0,0.0,0.0,0.0,0.0,...
                        t77.*(R.*t4.*w-R.*t4.*t9.*t10.*2.0+L.*R.*t14.*t18.*t23.*2.0+R.*kappa_1.*t19.*t20.*w+R.*t14.*t18.*t21.*w-R.*kappa_1.*t9.*t10.*t19.*t20.*2.0+L.*R.*kappa_2.*t4.*t18.*t22.*t26.*2.0-L.*R.*kappa_1.*t14.*t18.*t20.*t21.*2.0+L.*R.*kappa_2.*t18.*t22.*t23.*t25.*2.0+R.*kappa_2.*t4.*t18.*t22.*t27.*w+R.*kappa_1.*t14.*t18.*t20.*t23.*w+R.*kappa_2.*t18.*t21.*t22.*t25.*w+L.*R.*kappa_1.*kappa_2.*t18.*t19.*t20.*t22.*t26.*2.0-L.*R.*kappa_1.*kappa_2.*t18.*t20.*t21.*t22.*t25.*2.0+R.*kappa_1.*kappa_2.*t18.*t19.*t20.*t22.*t27.*w+R.*kappa_1.*kappa_2.*t18.*t20.*t22.*t23.*t25.*w), ...
                        t77.*(R.*t19.*w-R.*t9.*t10.*t19.*2.0+L.*R.*t18.*t23.*t28.*2.0-R.*kappa_1.*t4.*t20.*w+R.*t18.*t21.*t28.*w+R.*kappa_1.*t4.*t9.*t10.*t20.*2.0+L.*R.*kappa_2.*t18.*t19.*t22.*t26.*2.0-L.*R.*kappa_1.*t18.*t20.*t21.*t28.*2.0-L.*R.*kappa_2.*t18.*t22.*t23.*t31.*2.0+R.*kappa_2.*t18.*t19.*t22.*t27.*w+R.*kappa_1.*t18.*t20.*t23.*t28.*w-R.*kappa_2.*t18.*t21.*t22.*t31.*w-L.*R.*kappa_1.*kappa_2.*t4.*t18.*t20.*t22.*t26.*2.0+L.*R.*kappa_1.*kappa_2.*t18.*t20.*t21.*t22.*t31.*2.0-R.*kappa_1.*kappa_2.*t4.*t18.*t20.*t22.*t27.*w-R.*kappa_1.*kappa_2.*t18.*t20.*t22.*t23.*t31.*w), ...
                        R.*t18.*t77.*(t4.*t28-t14.*t19+kappa_1.*t4.*t14.*t20-kappa_2.*t4.*t22.*t31+kappa_1.*t19.*t20.*t28-kappa_2.*t19.*t22.*t25+kappa_1.*kappa_2.*t4.*t20.*t22.*t25-kappa_1.*kappa_2.*t19.*t20.*t22.*t31).*-2.0, ...
                        0.0, 0.0,t77.*(kappa_1.*t20+1.0).*(t106.*w+t107.*w-t9.*t10.*t106.*2.0-t9.*t10.*t107.*2.0+L.*t4.*t14.*t18.*t23.*2.0+L.*t4.*t18.*t21.*t28.*2.0-L.*t14.*t18.*t19.*t21.*2.0+L.*t18.*t19.*t23.*t28.*2.0+t4.*t14.*t18.*t21.*w-t4.*t18.*t23.*t28.*w+t14.*t18.*t19.*t23.*w+t18.*t19.*t21.*t28.*w+kappa_2.*t18.*t22.*t27.*t106.*w+kappa_2.*t18.*t22.*t27.*t107.*w+L.*kappa_2.*t18.*t22.*t26.*t106.*2.0+L.*kappa_2.*t18.*t22.*t26.*t107.*2.0+L.*kappa_2.*t4.*t18.*t22.*t23.*t25.*2.0-L.*kappa_2.*t4.*t18.*t21.*t22.*t31.*2.0-L.*kappa_2.*t18.*t19.*t21.*t22.*t25.*2.0-L.*kappa_2.*t18.*t19.*t22.*t23.*t31.*2.0+kappa_2.*t4.*t18.*t21.*t22.*t25.*w+kappa_2.*t4.*t18.*t22.*t23.*t31.*w+kappa_2.*t18.*t19.*t22.*t23.*t25.*w-kappa_2.*t18.*t19.*t21.*t22.*t31.*w), ...
                        1.0,0.0,0.0,0.0,0.0,0.0,0.0,0.0,0.0,0.0,L.*t7,1.0], ...
                        [9,3]);
